simulink model "lqr_zero_regulation_scheme"  (R2025b)
settings: Solver=VariableStepAuto  StartTime=0.0  StopTime=t_sim  RelTol=1e-3
values from neighbouring files (symbols this model uses):
  A = [0 1 ... (first row only)    [lqr_integral_tracking.m]    (also in lqr_zero_regulation.m = [0  1)
  B = [0 ... (first row only)    [lqr_integral_tracking.m]    (also in lqr_zero_regulation.m)
  C = [1 0]    [lqr_integral_tracking.m]    (also in lqr_zero_regulation.m)
  K = dlqr(Ad, Bd, Q, R)    [lqr_zero_regulation.m]
  Ts = 0.05    [lqr_integral_tracking.m]    (also in lqr_zero_regulation.m)
  x0 = [0.8; 0]    [lqr_integral_tracking.m]    (also in lqr_zero_regulation.m)
settings Model: Creator=nicol  LastModifiedBy=nicol

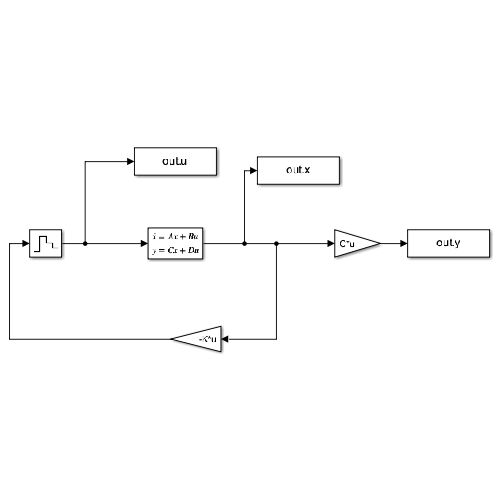
[thumbnail: Simulink's stored preview of the top-level diagram]
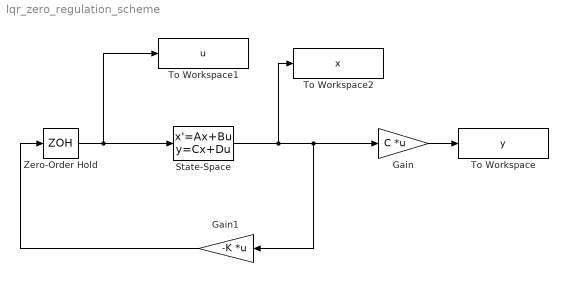
== system lqr_zero_regulation_scheme ==
  Gain : Gain  Gain=C  Multiplication=Matrix(K*u)
  Gain1 : Gain  Gain=-K  Multiplication=Matrix(K*u)
  State-Space : StateSpace  A=A  B=B  C=eye(2)  D=[0 ; 0]  InitialCondition=x0
  To Workspace : ToWorkspace  VariableName=y  SaveFormat=Timeseries  SampleTime=-1
  To Workspace1 : ToWorkspace  VariableName=u  SaveFormat=Timeseries  SampleTime=-1
  To Workspace2 : ToWorkspace  VariableName=x  SaveFormat=Timeseries  SampleTime=-1
  Zero-Order Hold : ZeroOrderHold  SampleTime=Ts
  wires:
  State-Space/1 -> To Workspace2/1, Gain1/1, Gain/1
  Gain/1 -> To Workspace/1
  Gain1/1 -> Zero-Order Hold/1
  Zero-Order Hold/1 -> State-Space/1, To Workspace1/1
